simulink library "tqd"  (R2021b)
settings: Solver=VariableStepAuto  StartTime=0.0  StopTime=10.0  RelTol=1e-3
undefined symbols (not defined in the file): ATQD_AfterTqMinGain_X_Deg, ATQD_APSCreepBaseTqD_X_kph, ATQD_APSCreepBaseTqD_Y_Deg, ATQD_APSCreepBaseTqR_X_kph, ATQD_APSCreepBaseTqR_Y_Deg, ATQD_APSCreepIterm_X_kph, ATQD_APSCreepIterm_Y_kph, ATQD_APSCreepPterm_X_kph, ATQD_APSCreepPterm_Y_kph, ATQD_APSDecReq_X_kph, ATQD_APSDecReq_Y_mps2, ATQD_APSDecReqCMD_X_kph, ATQD_APSDecReqTs_X_pct, ATQD_APSDecTimeGain_X_Deg, ATQD_APSDecTimeGain_Y_s, ATQD_APSReqLowSpd_X_Deg, ATQD_AutoHoldReleaseBPS_X_Deg, ATQD_AWDLoadTrqnsGain_X_kg, ATQD_AWDLoadTrqnsGain_Y_pct, ATQD_BOSEnBPSPosn_X_kph, ATQD_BOSMap_X_rpm, ATQD_BOSMap_Y_pct, ATQD_CreepBaseTqD_X_kph, ATQD_CreepBaseTqD_Y_Deg, ATQD_CreepBaseTqR_X_kph, ATQD_CreepBaseTqR_Y_Deg, ATQD_CreepBPSDisPosn_X_Deg, ATQD_CreepBPSDisPosnR_X_Deg, ATQD_CreepBPSEnPosn_X_Deg, ATQD_CreepBPSEnPosnR_X_Deg, ATQD_CreepDeltaTq_X_kph, ATQD_CreepIterm_X_kph, ATQD_CreepIterm_Y_kph, ATQD_CreepItermMaxLimit_X_pct, ATQD_CreepPreloadTime_X_kph, ATQD_CreepPreloadTq_X_kph, ATQD_CreepPreloadTq_Y_s, ATQD_CreepProtTq_X_Deg, ATQD_CreepPterm_X_kph, ATQD_CreepPterm_Y_kph, ATQD_CreepRrTqSpRat_X_rpm, ATQD_CreepRrTqSpRat_Y_Nm, ATQD_CreepTargetSpdD_X_pct, ATQD_CreepTargetSpdR_X_pct, ATQD_ECOTqMapD_X_rpm, ATQD_ECOTqMapD_Y_pct, ATQD_EMTqMapD_X_rpm, ATQD_EMTqMapD_Y_pct, ATQD_EOPDTqMapDCon_X_rpm, ATQD_EOPDTqMapDCon_Y_Deg, ATQD_EscapeModePedTq_X_pct, ATQD_EscapeModePedTq_Y_rpm, ATQD_EscapeModePedTqFr_X_pct, ATQD_EscapeModePedTqFr_Y_rpm, ATQD_EstInitVehWeight_X_c, ATQD_FAfterTqCMDGain_X_rpm, ATQD_FAfterTqCMDGain_Y_pct, ATQD_FrLossMAPLowV_X_rpm, ATQD_FrLossMAPLowV_Y_Nm, ATQD_FrMotActReduce_X_rpm ... (+772)
libraries: simulink x211, hcu_lib x179, tqr x3
(part 21 of 28)

== system tqd/TQD/TorqueDemand/TorqueModule/DriverWhlTqDem/PedalMapWhlTq/Pedal G-Control Mode/Torque Calculation ==
  VTQD_ActAPSPosn_pct : Inport
  VTQD_TqTargetShaftSpd_rpm : Inport  Port=2
  VVMC_LongAcc_Gps : Inport  Port=3
  VINP_VehSpeed_kph : Inport  Port=4
  VTQD_PedAccTqEn_flg : Inport  Port=5
  VTQD_GearActualPosn_enum : Inport  Port=6
  VTQD_CreepPrLoadEnable_flg : Inport  Port=7
  VINP_BrkPedalPos_pct : Inport  Port=8
  VINP_IVIPedalGRegenLim_pct : Inport  Port=9
  VVMC_SmartRegenReq_mps2 : Inport  Port=10
  VINP_IVISmartRegenSW_flg : Inport  Port=11
  VINP_IVICreepOnSW_flg : Inport  Port=12
  VTQD_APSReqTimer_s : Inport  Port=13
  AND{,1..3} (4 alike) : Logic  AllPortsSameDT=off  OutDataTypeStr=boolean
  Add : Sum
  Add1 : Sum  Inputs=+-
  Constant1 : Constant  Value=KTQD_PedAccCMDUpLim_mps2
  Constant10 : Constant  Value=KVMC_GravityValue_mps2
  Constant11 : Constant  Value=KTQD_PedAccDevLowLim_mps2
  Constant12 : Constant  Value=ONE_PERCENT
  Constant13 : Constant  Value=KTQD_PedAccBrkEnPos_pct
  Constant14 : Constant  Value=KTQD_PedAccBrkDeltaTq_Nm
  Constant{6..7,15,21} (4 alike) : Constant  Value=ZERO_INT
  Constant16 : Constant  Value=ZERO_FLOAT
  Constant17 : Constant  Value=KTQD_PedAccARgnEnSpd_kph
  Constant18 : Constant  Value=KTQD_PedAccBrkEnPos_pct
  Constant19 : Constant  Value=KTQD_PedAccDevUpLim_mps2
  Constant2 : Constant  Value=KTQD_PedAccCMDLowLim_mps2
  Constant20 : Constant  Value=KTQD_PedAccARgnEnSpd_kph
  Constant22 : Constant  Value=KTQD_APSReqDelayTime_s
  Constant23 : Constant  Value=KTQD_PedAccCMDLowLim_mps2
  Constant3 : Constant  Value=KTQD_PedAccTqUpLim_Nm
  Constant4 : Constant  Value=KTQD_PedAccTqLowLim_Nm
  Constant5 : Constant  Value=KTQD_PedGControlEnSpd_kph
  Constant8 : Constant  Value=ENUM_GEARACTUALPOSN_D
  Constant9 : Constant  Value=ZERO_FLOAT
  Delay : Delay  DelayLength=1
  Delay1 : Delay  DelayLength=1
  Equal : RelationalOperator  Operator===  OutDataTypeStr=boolean  RndMeth=Simplest
  Equal1 : RelationalOperator  OutDataTypeStr=boolean  RndMeth=Simplest
  MTQD_PedAccBrkTq_Y_Nm : Lookup_n-D  NumberOfTableDimensions=1  BreakpointsForDimension1=ATQD_PedAccBrkTq_X_pct  Table=MTQD_PedAccBrkTq_Y_Nm  InternalRulePriority=Speed  RndMeth=Simplest  InputSameDT=on
  MTQD_PedalAccelCMDWC_Z_mps2 : Lookup_n-D  BreakpointsForDimension1=ATQD_PedalAccelCMD_Y_pct  BreakpointsForDimension2=ATQD_PedalAccelCMD_X_rpm  BreakpointsForDimension3=[5, 7]  Table=MTQD_PedalAccelCMDWC_Z_mps2  ExtrapMethod=Clip  InternalRulePriority=Speed  RndMeth=Simplest  InputSameDT=on
      settings: InputPortMap=u0,u1
  MTQD_PedalAccelCMD_Z_mps2 : Lookup_n-D  BreakpointsForDimension1=ATQD_PedalAccelCMD_Y_pct  BreakpointsForDimension2=ATQD_PedalAccelCMD_X_rpm  BreakpointsForDimension3=[5, 7]  Table=MTQD_PedalAccelCMD_Z_mps2  ExtrapMethod=Clip  InternalRulePriority=Speed  RndMeth=Simplest  InputSameDT=on
      settings: InputPortMap=u0,u1
  MTQD_PedalGDeltaTqIGain_Z_Nm : Lookup_n-D  BreakpointsForDimension1=ATQD_PedalGDeltaTqIGain_Y_mps2  BreakpointsForDimension2=ATQD_PedalGDeltaTqIGain_X_kph  Table=MTQD_PedalGDeltaTqIGain_Z_Nm  InternalRulePriority=Speed  RndMeth=Simplest  InputSameDT=on
      settings: InputPortMap=u0,u1
  Max : MinMax  Function=max  Inputs=2
  OR : Logic  Operator=OR  AllPortsSameDT=off  OutDataTypeStr=boolean
  OR1 : Logic  Operator=OR  AllPortsSameDT=off  OutDataTypeStr=boolean
  Product : Product
  Product1 : Product  Inputs=3
  Relational Operator : RelationalOperator  Operator=<=  OutDataTypeStr=boolean  RndMeth=Simplest
  Relational Operator1 : RelationalOperator  Operator=<=  OutDataTypeStr=boolean  RndMeth=Simplest
  Relational Operator3 : RelationalOperator  OutDataTypeStr=boolean  RndMeth=Simplest
  Relational Operator4 : RelationalOperator  OutDataTypeStr=boolean  RndMeth=Simplest
  Relational Operator5 : RelationalOperator  Operator=>  OutDataTypeStr=boolean  RndMeth=Simplest
  Relational Operator6 : RelationalOperator  OutDataTypeStr=boolean  RndMeth=Simplest
  Relational Operator7 : RelationalOperator  Operator=<=  OutDataTypeStr=boolean  RndMeth=Simplest
  Saturation Dynamic{,1..3} (4 alike) : simulink/Discontinuities/Saturation Dynamic  OutMin=[]  OutMax=[]  OutDataTypeStr=Inherit: Same as second input  OutDataType=fixdt(1, 16)  OutScaling=2^-10  DoSatur=off
  Switch{,1..6} (7 alike) : Switch  Criteria=u2 > Threshold
  VTQD_PedalTqCal_Nm : Outport
  wires:
  Saturation Dynamic1/1 -> MTQD_PedalGDeltaTqIGain_Z_Nm/1  "VTQD_PedalAccDev_mps2"
  [VTQD_PedalAccDeltaTq_Nm] -> Add/1
  Constant11/1 -> Saturation Dynamic1/3
  [VTQD_PedalReqAccel_mps2] -> Add1/1
  [VTQD_ActAPSPosn_pct] -> MTQD_PedalAccelCMD_Z_mps2/1
  [VTQD_TqTargetShaftSpd_rpm] -> MTQD_PedalAccelCMD_Z_mps2/2
  Constant6/1 -> Switch/3
  [VVMC_LongAcc_Gps] -> Product/1
  [VINP_VehSpeed_kph] -> MTQD_PedalGDeltaTqIGain_Z_Nm/2
  Add1/1 -> Saturation Dynamic1/2
  Constant19/1 -> Saturation Dynamic1/1
  Constant10/1 -> Product/2
  Constant1/1 -> Saturation Dynamic2/1
  Delay/1 -> [VTQD_LastPedalTqCal_Nm]  "VTQD_LastPedalTqCal_Nm"
  Product/1 -> Add1/2
  Switch/1 -> Saturation Dynamic/2
  Saturation Dynamic2/1 -> [VTQD_PedalReqAccel_mps2]  "VTQD_PedalReqAccel_mps2"
  [VTQD_LastPedalTqCal_Nm] -> Add/2
  VTQD_ActAPSPosn_pct/1 -> [VTQD_ActAPSPosn_pct]
  VTQD_TqTargetShaftSpd_rpm/1 -> [VTQD_TqTargetShaftSpd_rpm]
  VVMC_LongAcc_Gps/1 -> [VVMC_LongAcc_Gps]
  VINP_VehSpeed_kph/1 -> [VINP_VehSpeed_kph]
  VTQD_PedAccTqEn_flg/1 -> [VTQD_PedAccTqEn_flg]
  [VTQD_PedalTqCal_Nm] -> VTQD_PedalTqCal_Nm/1
  [VINP_VehSpeed_kph] -> Relational Operator/1
  Constant5/1 -> Relational Operator/2
  Relational Operator/1 -> AND/1
  Constant4/1 -> Switch1/3
  Constant7/1 -> Switch1/1
  Switch1/1 -> [VTQD_PedAccTqLowLim_Nm]  "VTQD_PedAccTqLowLim_Nm"
  [VTQD_PedAccTqLowLim_Nm] -> Saturation Dynamic/3
  [VTQD_PedAccTqEn_flg] -> AND1/1
  Equal/1 -> AND1/2
  [VTQD_GearActualPosn_enum] -> Equal/1
  Constant8/1 -> Equal/2
  VTQD_GearActualPosn_enum/1 -> [VTQD_GearActualPosn_enum]
  VTQD_CreepPrLoadEnable_flg/1 -> [VTQD_CreepPrLoadEnable_flg]
  Add/1 -> Switch/1
  [VTQD_PedalReqAccel_mps2] -> Relational Operator1/1
  Relational Operator1/1 -> AND/2
  Constant9/1 -> Relational Operator1/2
  AND/1 -> OR1/1
  OR1/1 -> Switch1/2
  Delay1/1 -> OR1/2
  [VTQD_CreepPrLoadEnable_flg] -> Delay1/1
  VINP_BrkPedalPos_pct/1 -> [VINP_BrkPedalPos_pct]
  [VINP_BrkPedalPos_pct] -> Relational Operator3/1
  Constant13/1 -> Relational Operator3/2
  Switch3/1 -> Switch2/1
  Constant14/1 -> Switch3/1
  [VTQD_LastPedalTqCal_Nm] -> Relational Operator4/1
  Relational Operator4/1 -> Switch3/2
  Constant16/1 -> Switch3/3
  Saturation Dynamic/1 -> [VTQD_PedalTqCal_Nm], Delay/1  "VTQD_PedalTqCal_Nm"
  MTQD_PedalGDeltaTqIGain_Z_Nm/1 -> Switch2/3
  Switch2/1 -> [VTQD_PedalAccDeltaTq_Nm]  "VTQD_PedalAccDeltaTq_Nm"
  AND2/1 -> Switch2/2
  Relational Operator3/1 -> AND2/1
  [VINP_VehSpeed_kph] -> Relational Operator5/1
  Constant17/1 -> Relational Operator5/2
  Relational Operator5/1 -> AND2/2
  Relational Operator7/1 -> AND3/2
  Constant20/1 -> Relational Operator7/2
  [VINP_BrkPedalPos_pct] -> Relational Operator6/1
  Constant18/1 -> Relational Operator6/2
  [VINP_VehSpeed_kph] -> Relational Operator7/1
  Relational Operator6/1 -> AND3/1
  AND3/1 -> Switch4/2
  Constant3/1 -> Switch4/3
  Constant21/1 -> Switch4/1
  Switch4/1 -> [VTQD_PedAccTqUpLim_Nm]  "VTQD_PedAccTqUpLim_Nm"
  [VTQD_PedAccTqUpLim_Nm] -> Saturation Dynamic/1
  [VTQD_PedAccBrkTq_Nm] -> Relational Operator4/2
  MTQD_PedAccBrkTq_Y_Nm/1 -> Saturation Dynamic3/2
  Saturation Dynamic3/1 -> [VTQD_PedAccBrkTq_Nm]  "VTQD_PedAccBrkTq_Nm"
  Constant15/1 -> Saturation Dynamic3/1
  [VTQD_PedAccTqLowLim_Nm] -> Saturation Dynamic3/3
  VINP_IVIPedalGRegenLim_pct/1 -> [VINP_IVIPedalGRegenLim_pct]
  [VINP_IVIPedalGRegenLim_pct] -> MTQD_PedAccBrkTq_Y_Nm/1
  Constant2/1 -> Product1/1
  [VINP_IVIPedalGRegenLim_pct] -> Product1/2
  Constant12/1 -> Product1/3
  Product1/1 -> Max/1
  Max/1 -> Saturation Dynamic2/3
  Switch5/1 -> Max/2
  [VVMC_SmartRegenReq_mps2] -> Switch5/1
  Constant23/1 -> Switch5/3
  [VINP_IVISmartRegenSW_flg] -> Switch5/2
  VVMC_SmartRegenReq_mps2/1 -> [VVMC_SmartRegenReq_mps2]
  VINP_IVISmartRegenSW_flg/1 -> [VINP_IVISmartRegenSW_flg]
  MTQD_PedalAccelCMD_Z_mps2/1 -> [VTQD_PedalAccelCMD_mps2]  "VTQD_PedalAccelCMD_mps2"
  MTQD_PedalAccelCMDWC_Z_mps2/1 -> [VTQD_PedalAccelCMDWC_mps2]  "VTQD_PedalAccelCMDWC_mps2"
  [VTQD_TqTargetShaftSpd_rpm] -> MTQD_PedalAccelCMDWC_Z_mps2/2
  [VTQD_ActAPSPosn_pct] -> MTQD_PedalAccelCMDWC_Z_mps2/1
  VINP_IVICreepOnSW_flg/1 -> [VINP_IVICreepOnSW_flg]
  Switch6/1 -> Saturation Dynamic2/2
  [VINP_IVICreepOnSW_flg] -> Switch6/2
  [VTQD_PedalAccelCMD_mps2] -> Switch6/3
  [VTQD_PedalAccelCMDWC_mps2] -> Switch6/1
  VTQD_APSReqTimer_s/1 -> [VTQD_APSReqTimer_s]
  OR/1 -> Switch/2
  AND1/1 -> OR/1
  Equal1/1 -> OR/2
  [VTQD_APSReqTimer_s] -> Equal1/1
  Constant22/1 -> Equal1/2

== system tqd/TQD/TorqueDemand/Signal_convert/SWC2_Subsystem/Big Mike Combo/Combo Key Detection/DiagnosisOff Mode/Key1 ==
  VSCP_ComboKeyCMD_enum : Inport
  VSCP_ComboKeyEn_flg : Inport  Port=2
  VSCP_ComboKeyReset_flg : Inport  Port=3
  AND : Logic  Inputs=3  AllPortsSameDT=off  OutDataTypeStr=boolean
  Constant1 : Constant  Value=KTQD_DiagnosisOff1_enum
  Constant2 : Constant  Value=ENUM_COMBOKEY_NONE
  Constant4 : Constant  Value=ENUM_COMBOKEY_NONE
  Data Type Conversion : DataTypeConversion  OutDataTypeStr=uint8
  Delay : Delay  DelayLength=1
  Delay1 : Delay  DelayLength=1
  Detect Change : simulink/Logic and Bit Operations/Detect Change  vinit=0  OutDataTypeStr=boolean
  Detect Increase : simulink/Logic and Bit Operations/Detect Increase  vinit=0.0  OutDataTypeStr=boolean
  Equal : RelationalOperator  Operator===  OutDataTypeStr=boolean  RndMeth=Simplest
  Equal1 : RelationalOperator  Operator=~=  OutDataTypeStr=boolean  RndMeth=Simplest
  Equal2 : RelationalOperator  Operator===  OutDataTypeStr=boolean  RndMeth=Simplest
  If : If  NumInputs=2  IfExpression=u1 ~=0  ElseIfExpressions=u2 ~= 0
  Maintain : Subsystem  TreatAsAtomicUnit=on
  Merge : Merge  Inputs=3
  OR : Logic  Operator=OR  AllPortsSameDT=off  OutDataTypeStr=boolean
  Reset : Subsystem  TreatAsAtomicUnit=on
  Write : Subsystem  TreatAsAtomicUnit=on
  VSCP_ComboKey1_enum : Outport
  VSCP_Key1Pass_flg : Outport  Port=2
  wires:
  Data Type Conversion/1 -> [VSCP_ComboKey1_enum]  "VTQD_DiagnosisOff1_enum"
  Delay1/1 -> Maintain/1(Input)
  [VSCP_ComboKey1_enum] -> Delay1/1
  [VSCP_Key1Pass_flg] -> VSCP_Key1Pass_flg/1
  [VSCP_ComboKey1_enum] -> VSCP_ComboKey1_enum/1
  VSCP_ComboKeyEn_flg/1 -> [VSCP_ComboKeyEn_flg]
  VSCP_ComboKeyReset_flg/1 -> [VSCP_ComboKeyReset_flg]
  VSCP_ComboKeyCMD_enum/1 -> [VSCP_ComboKeyCMD_enum]
  Equal/1 -> [VSCP_Key1Pass_flg]  "VTQD_DiagnosisOff1Pass_flg"
  Constant1/1 -> Equal/2
  [VSCP_ComboKey1_enum] -> Equal/1
  If/2 -> Write/Action
  Write/1(WriteCMD) -> Merge/2
  If/1 -> Reset/Action
  Detect Increase/1 -> OR/1
  AND/1 -> [VSCP_WriteComboCMD_flg]  "VSCP_WriteComboCMD_flg"
  [VSCP_ComboKeyCMD_enum] -> Write/1(Input)
  [VSCP_ComboKeyCMD_enum] -> Detect Change/1
  [VSCP_ResetComboKey_flg] -> If/1
  [VSCP_ComboKeyEn_flg] -> Detect Increase/1
  Detect Change/1 -> AND/1
  Maintain/1(KeepKey1) -> Merge/3
  Constant4/1 -> Equal1/2
  If/3 -> Maintain/Action
  Delay/1 -> Equal2/1
  Merge/1 -> Data Type Conversion/1
  Reset/1(ResetToZero) -> Merge/1
  Equal2/1 -> AND/3
  Constant2/1 -> Equal2/2
  Equal1/1 -> AND/2
  [VSCP_ComboKey1_enum] -> Delay/1
  [VSCP_ComboKeyReset_flg] -> OR/2
  [VSCP_ComboKeyCMD_enum] -> Equal1/1
  [VSCP_WriteComboCMD_flg] -> If/2
  OR/1 -> [VSCP_ResetComboKey_flg]  "VSCP_ResetComboKey_flg"

== system tqd/TQD/TorqueDemand/Signal_convert/SWC2_Subsystem/Big Mike Combo/Combo Key Detection/DiagnosisOff Mode/Key2 ==
  VSCP_ComboKeyCMD_enum : Inport
  VSCP_ComboKeyEn_flg : Inport  Port=2
  VSCP_ComboKeyReset_flg : Inport  Port=3
  VSCP_ComboKey1_enum : Inport  Port=4
  AND : Logic  Inputs=4  AllPortsSameDT=off  OutDataTypeStr=boolean
  Constant1 : Constant  Value=KTQD_DiagnosisOff2_enum
  Constant2 : Constant  Value=ENUM_COMBOKEY_NONE
  Constant3 : Constant  Value=ENUM_COMBOKEY_NONE
  Constant4 : Constant  Value=ENUM_COMBOKEY_NONE  OutDataTypeStr=uint8
  Data Type Conversion : DataTypeConversion  OutDataTypeStr=uint8
  Delay : Delay  DelayLength=1
  Delay1 : Delay  DelayLength=1
  Delay2 : Delay  DelayLength=1
  Detect Change : simulink/Logic and Bit Operations/Detect Change  vinit=0  OutDataTypeStr=boolean
  Detect Increase : simulink/Logic and Bit Operations/Detect Increase  vinit=0.0  OutDataTypeStr=boolean
  Equal : RelationalOperator  Operator===  OutDataTypeStr=boolean  RndMeth=Simplest
  Equal1 : RelationalOperator  Operator=~=  OutDataTypeStr=boolean  RndMeth=Simplest
  Equal2 : RelationalOperator  Operator=~=  OutDataTypeStr=boolean  RndMeth=Simplest
  Equal3 : RelationalOperator  Operator===  OutDataTypeStr=boolean  RndMeth=Simplest
  If : If  NumInputs=2  IfExpression=u1 ~=0  ElseIfExpressions=u2 ~= 0
  Maintain : Subsystem  TreatAsAtomicUnit=on
  Merge : Merge  Inputs=3
  OR : Logic  Operator=OR  AllPortsSameDT=off  OutDataTypeStr=boolean
  Reset : Subsystem  TreatAsAtomicUnit=on
  Write : Subsystem  TreatAsAtomicUnit=on
  VSCP_ComboKey2_enum : Outport
  VSCP_Key2Pass_flg : Outport  Port=2
  wires:
  Data Type Conversion/1 -> [VSCP_ComboKey2_enum]  "VTQD_DiagnosisOff2_enum"
  [VSCP_ComboKey2_enum] -> Delay2/1
  Delay2/1 -> Maintain/1(Input)
  Equal3/1 -> AND/4
  Delay1/1 -> Equal3/1
  Constant3/1 -> Equal3/2
  [VSCP_ComboKey2_enum] -> Delay1/1
  VSCP_ComboKey1_enum/1 -> [VSCP_ComboKey1_enum]
  OR/1 -> [VSCP_ResetComboKey_flg]  "VSCP_ResetComboKey_flg"
  [VSCP_WriteComboCMD_flg] -> If/2
  [VSCP_ComboKeyCMD_enum] -> Equal1/1
  [VSCP_ComboKeyReset_flg] -> OR/2
  [VSCP_ComboKey1_enum] -> Delay/1
  Equal1/1 -> AND/2
  Constant2/1 -> Equal2/2
  Equal2/1 -> AND/3
  Reset/1(ResetToZero) -> Merge/1
  Merge/1 -> Data Type Conversion/1
  Delay/1 -> Equal2/1
  If/3 -> Maintain/Action
  Constant4/1 -> Equal1/2
  Maintain/1(KeepKey2) -> Merge/3
  Detect Change/1 -> AND/1
  [VSCP_ComboKeyEn_flg] -> Detect Increase/1
  [VSCP_ResetComboKey_flg] -> If/1
  [VSCP_ComboKeyCMD_enum] -> Detect Change/1
  [VSCP_ComboKeyCMD_enum] -> Write/1(Input)
  AND/1 -> [VSCP_WriteComboCMD_flg]  "VSCP_WriteComboCMD_flg"
  Detect Increase/1 -> OR/1
  If/1 -> Reset/Action
  Write/1(WriteCMD) -> Merge/2
  If/2 -> Write/Action
  [VSCP_ComboKey2_enum] -> Equal/1
  Constant1/1 -> Equal/2
  Equal/1 -> [VSCP_Key2Pass_flg]  "VTQD_DiagnosisOff2Pass_flg"
  VSCP_ComboKeyCMD_enum/1 -> [VSCP_ComboKeyCMD_enum]
  VSCP_ComboKeyReset_flg/1 -> [VSCP_ComboKeyReset_flg]
  VSCP_ComboKeyEn_flg/1 -> [VSCP_ComboKeyEn_flg]
  [VSCP_ComboKey2_enum] -> VSCP_ComboKey2_enum/1
  [VSCP_Key2Pass_flg] -> VSCP_Key2Pass_flg/1

== system tqd/TQD/TorqueDemand/Signal_convert/SWC2_Subsystem/Big Mike Combo/Combo Key Detection/DiagnosisOff Mode/Key3 ==
  VSCP_ComboKeyCMD_enum : Inport
  VSCP_ComboKeyEn_flg : Inport  Port=2
  VSCP_ComboKeyReset_flg : Inport  Port=3
  VSCP_ComboKey2_enum : Inport  Port=4
  AND : Logic  Inputs=4  AllPortsSameDT=off  OutDataTypeStr=boolean
  Constant1 : Constant  Value=KTQD_DiagnosisOff3_enum
  Constant2 : Constant  Value=ENUM_COMBOKEY_NONE
  Constant3 : Constant  Value=ENUM_COMBOKEY_NONE
  Constant4 : Constant  Value=ENUM_COMBOKEY_NONE
  Data Type Conversion : DataTypeConversion  OutDataTypeStr=uint8
  Delay : Delay  DelayLength=1
  Delay1 : Delay  DelayLength=1
  Delay2 : Delay  DelayLength=1
  Detect Change : simulink/Logic and Bit Operations/Detect Change  vinit=0  OutDataTypeStr=boolean
  Detect Increase : simulink/Logic and Bit Operations/Detect Increase  vinit=0.0  OutDataTypeStr=boolean
  Equal : RelationalOperator  Operator===  OutDataTypeStr=boolean  RndMeth=Simplest
  Equal1 : RelationalOperator  Operator=~=  OutDataTypeStr=boolean  RndMeth=Simplest
  Equal2 : RelationalOperator  Operator=~=  OutDataTypeStr=boolean  RndMeth=Simplest
  Equal3 : RelationalOperator  Operator===  OutDataTypeStr=boolean  RndMeth=Simplest
  If : If  NumInputs=2  IfExpression=u1 ~=0  ElseIfExpressions=u2 ~= 0
  Maintain : Subsystem  TreatAsAtomicUnit=on
  Merge : Merge  Inputs=3
  OR : Logic  Operator=OR  AllPortsSameDT=off  OutDataTypeStr=boolean
  Reset : Subsystem  TreatAsAtomicUnit=on
  Write : Subsystem  TreatAsAtomicUnit=on
  VSCP_ComboKey3_enum : Outport
  VSCP_Key3Pass_flg : Outport  Port=2
  wires:
  Data Type Conversion/1 -> [VSCP_ComboKey3_enum]  "VTQD_DiagnosisOff3_enum"
  [VSCP_ComboKey3_enum] -> Delay2/1
  Delay2/1 -> Maintain/1(Input)
  [VSCP_ComboKey3_enum] -> Delay1/1
  Constant3/1 -> Equal3/2
  Equal3/1 -> AND/4
  Delay1/1 -> Equal3/1
  [VSCP_Key3Pass_flg] -> VSCP_Key3Pass_flg/1
  [VSCP_ComboKey3_enum] -> Equal/1
  [VSCP_ComboKey3_enum] -> VSCP_ComboKey3_enum/1
  VSCP_ComboKeyEn_flg/1 -> [VSCP_ComboKeyEn_flg]
  VSCP_ComboKeyReset_flg/1 -> [VSCP_ComboKeyReset_flg]
  VSCP_ComboKeyCMD_enum/1 -> [VSCP_ComboKeyCMD_enum]
  Equal/1 -> [VSCP_Key3Pass_flg]  "VTQD_DiagnosisOff3Pass_flg"
  Constant1/1 -> Equal/2
  If/2 -> Write/Action
  Write/1(WriteCMD) -> Merge/2
  If/1 -> Reset/Action
  Detect Increase/1 -> OR/1
  AND/1 -> [VSCP_WriteComboCMD_flg]  "VSCP_WriteComboCMD_flg"
  [VSCP_ComboKeyCMD_enum] -> Write/1(Input)
  [VSCP_ComboKeyCMD_enum] -> Detect Change/1
  [VSCP_ResetComboKey_flg] -> If/1
  [VSCP_ComboKeyEn_flg] -> Detect Increase/1
  Detect Change/1 -> AND/1
  Maintain/1(KeepKey3) -> Merge/3
  Constant4/1 -> Equal1/2
  If/3 -> Maintain/Action
  Delay/1 -> Equal2/1
  Merge/1 -> Data Type Conversion/1
  Reset/1(ResetToZero) -> Merge/1
  Equal2/1 -> AND/3
  Constant2/1 -> Equal2/2
  Equal1/1 -> AND/2
  [VSCP_ComboKey2_enum] -> Delay/1
  [VSCP_ComboKeyReset_flg] -> OR/2
  [VSCP_ComboKeyCMD_enum] -> Equal1/1
  [VSCP_WriteComboCMD_flg] -> If/2
  OR/1 -> [VSCP_ResetComboKey_flg]  "VSCP_ResetComboKey_flg"
  VSCP_ComboKey2_enum/1 -> [VSCP_ComboKey2_enum]

== system tqd/TQD/TorqueDemand/Signal_convert/SWC2_Subsystem/Big Mike Combo/Combo Key Detection/DiagnosisOff Mode/Key4 ==
  VSCP_ComboKeyCMD_enum : Inport
  VSCP_ComboKeyEn_flg : Inport  Port=2
  VSCP_ComboKeyReset_flg : Inport  Port=3
  VSCP_ComboKey3_enum : Inport  Port=4
  AND : Logic  Inputs=4  AllPortsSameDT=off  OutDataTypeStr=boolean
  Constant1 : Constant  Value=KTQD_DiagnosisOff4_enum
  Constant2 : Constant  Value=ENUM_COMBOKEY_NONE
  Constant3 : Constant  Value=ENUM_COMBOKEY_NONE
  Constant4 : Constant  Value=ENUM_COMBOKEY_NONE
  Data Type Conversion : DataTypeConversion  OutDataTypeStr=uint8
  Delay : Delay  DelayLength=1
  Delay1 : Delay  DelayLength=1
  Delay2 : Delay  DelayLength=1
  Detect Change : simulink/Logic and Bit Operations/Detect Change  vinit=0  OutDataTypeStr=boolean
  Detect Increase : simulink/Logic and Bit Operations/Detect Increase  vinit=0.0  OutDataTypeStr=boolean
  Equal : RelationalOperator  Operator===  OutDataTypeStr=boolean  RndMeth=Simplest
  Equal1 : RelationalOperator  Operator=~=  OutDataTypeStr=boolean  RndMeth=Simplest
  Equal2 : RelationalOperator  Operator=~=  OutDataTypeStr=boolean  RndMeth=Simplest
  Equal3 : RelationalOperator  Operator===  OutDataTypeStr=boolean  RndMeth=Simplest
  If : If  NumInputs=2  IfExpression=u1 ~=0  ElseIfExpressions=u2 ~= 0
  Maintain : Subsystem  TreatAsAtomicUnit=on
  Merge : Merge  Inputs=3
  OR : Logic  Operator=OR  AllPortsSameDT=off  OutDataTypeStr=boolean
  Reset : Subsystem  TreatAsAtomicUnit=on
  Write : Subsystem  TreatAsAtomicUnit=on
  VSCP_ComboKey4_enum : Outport
  VSCP_Key4Pass_flg : Outport  Port=2
  wires:
  Data Type Conversion/1 -> [VSCP_ComboKey4_enum]  "VTQD_DiagnosisOff4_enum"
  Delay2/1 -> Maintain/1(Input)
  [VSCP_ComboKey4_enum] -> Delay2/1
  [VSCP_ComboKey4_enum] -> VSCP_ComboKey4_enum/1
  [VSCP_Key4Pass_flg] -> VSCP_Key4Pass_flg/1
  Equal3/1 -> AND/4
  Delay1/1 -> Equal3/1
  Constant3/1 -> Equal3/2
  [VSCP_ComboKey4_enum] -> Delay1/1
  VSCP_ComboKey3_enum/1 -> [VSCP_ComboKey3_enum]
  OR/1 -> [VSCP_ResetComboKey_flg]  "VSCP_ResetComboKey_flg"
  [VSCP_WriteComboCMD_flg] -> If/2
  [VSCP_ComboKeyCMD_enum] -> Equal1/1
  [VSCP_ComboKeyReset_flg] -> OR/2
  [VSCP_ComboKey3_enum] -> Delay/1
  Equal1/1 -> AND/2
  Constant2/1 -> Equal2/2
  Equal2/1 -> AND/3
  Reset/1(ResetToZero) -> Merge/1
  Merge/1 -> Data Type Conversion/1
  Delay/1 -> Equal2/1
  If/3 -> Maintain/Action
  Constant4/1 -> Equal1/2
  Maintain/1(KeepKey4) -> Merge/3
  Detect Change/1 -> AND/1
  [VSCP_ComboKeyEn_flg] -> Detect Increase/1
  [VSCP_ResetComboKey_flg] -> If/1
  [VSCP_ComboKeyCMD_enum] -> Detect Change/1
  [VSCP_ComboKeyCMD_enum] -> Write/1(Input)
  AND/1 -> [VSCP_WriteComboCMD_flg]  "VSCP_WriteComboCMD_flg"
  Detect Increase/1 -> OR/1
  If/1 -> Reset/Action
  Write/1(WriteCMD) -> Merge/2
  If/2 -> Write/Action
  Constant1/1 -> Equal/2
  Equal/1 -> [VSCP_Key4Pass_flg]  "VTQD_DiagnosisOff4Pass_flg"
  VSCP_ComboKeyCMD_enum/1 -> [VSCP_ComboKeyCMD_enum]
  VSCP_ComboKeyReset_flg/1 -> [VSCP_ComboKeyReset_flg]
  VSCP_ComboKeyEn_flg/1 -> [VSCP_ComboKeyEn_flg]
  [VSCP_ComboKey4_enum] -> Equal/1

== system tqd/TQD/TorqueDemand/Signal_convert/SWC2_Subsystem/Big Mike Combo/Combo Key Detection/DiagnosisOff Mode/Key5 ==
  VSCP_ComboKeyCMD_enum : Inport
  VSCP_ComboKeyEn_flg : Inport  Port=2
  VSCP_ComboKeyReset_flg : Inport  Port=3
  VSCP_ComboKey4_enum : Inport  Port=4
  AND : Logic  Inputs=4  AllPortsSameDT=off  OutDataTypeStr=boolean
  Constant1 : Constant  Value=KTQD_DiagnosisOff5_enum
  Constant2 : Constant  Value=ENUM_COMBOKEY_NONE
  Constant3 : Constant  Value=ENUM_COMBOKEY_NONE
  Constant4 : Constant  Value=ENUM_COMBOKEY_NONE
  Data Type Conversion : DataTypeConversion  OutDataTypeStr=uint8
  Delay : Delay  DelayLength=1
  Delay1 : Delay  DelayLength=1
  Delay2 : Delay  DelayLength=1
  Detect Change : simulink/Logic and Bit Operations/Detect Change  vinit=0  OutDataTypeStr=boolean
  Detect Increase : simulink/Logic and Bit Operations/Detect Increase  vinit=0.0  OutDataTypeStr=boolean
  Equal : RelationalOperator  Operator===  OutDataTypeStr=boolean  RndMeth=Simplest
  Equal1 : RelationalOperator  Operator=~=  OutDataTypeStr=boolean  RndMeth=Simplest
  Equal2 : RelationalOperator  Operator=~=  OutDataTypeStr=boolean  RndMeth=Simplest
  Equal3 : RelationalOperator  Operator===  OutDataTypeStr=boolean  RndMeth=Simplest
  If : If  NumInputs=2  IfExpression=u1 ~=0  ElseIfExpressions=u2 ~= 0
  Maintain : Subsystem  TreatAsAtomicUnit=on
  Merge : Merge  Inputs=3
  OR : Logic  Operator=OR  AllPortsSameDT=off  OutDataTypeStr=boolean
  Reset : Subsystem  TreatAsAtomicUnit=on
  Write : Subsystem  TreatAsAtomicUnit=on
  VSCP_ComboKey5_enum : Outport
  VSCP_Key5Pass_flg : Outport  Port=2
  wires:
  Data Type Conversion/1 -> [VSCP_ComboKey5_enum]  "VTQD_DiagnosisOff5_enum"
  Delay2/1 -> Maintain/1(Input)
  [VSCP_ComboKey5_enum] -> Delay2/1
  [VSCP_ComboKey5_enum] -> VSCP_ComboKey5_enum/1
  [VSCP_ComboKey5_enum] -> Equal/1
  VSCP_ComboKeyEn_flg/1 -> [VSCP_ComboKeyEn_flg]
  VSCP_ComboKeyReset_flg/1 -> [VSCP_ComboKeyReset_flg]
  VSCP_ComboKeyCMD_enum/1 -> [VSCP_ComboKeyCMD_enum]
  Equal/1 -> [VSCP_Key5Pass_flg]  "VTQD_DiagnosisOff5Pass_flg"
  Constant1/1 -> Equal/2
  If/2 -> Write/Action
  Write/1(WriteCMD) -> Merge/2
  If/1 -> Reset/Action
  Detect Increase/1 -> OR/1
  AND/1 -> [VSCP_WriteComboCMD_flg]  "VSCP_WriteComboCMD_flg"
  [VSCP_ComboKeyCMD_enum] -> Write/1(Input)
  [VSCP_ComboKeyCMD_enum] -> Detect Change/1
  [VSCP_ResetComboKey_flg] -> If/1
  [VSCP_ComboKeyEn_flg] -> Detect Increase/1
  Detect Change/1 -> AND/1
  Maintain/1(KeepKey5) -> Merge/3
  Constant4/1 -> Equal1/2
  If/3 -> Maintain/Action
  Delay/1 -> Equal2/1
  Merge/1 -> Data Type Conversion/1
  Reset/1(ResetToZero) -> Merge/1
  Equal2/1 -> AND/3
  Constant2/1 -> Equal2/2
  Equal1/1 -> AND/2
  [VSCP_ComboKey4_enum] -> Delay/1
  [VSCP_ComboKeyReset_flg] -> OR/2
  [VSCP_ComboKeyCMD_enum] -> Equal1/1
  [VSCP_WriteComboCMD_flg] -> If/2
  OR/1 -> [VSCP_ResetComboKey_flg]  "VSCP_ResetComboKey_flg"
  VSCP_ComboKey4_enum/1 -> [VSCP_ComboKey4_enum]
  [VSCP_ComboKey5_enum] -> Delay1/1
  Constant3/1 -> Equal3/2
  Delay1/1 -> Equal3/1
  Equal3/1 -> AND/4
  [VSCP_Key5Pass_flg] -> VSCP_Key5Pass_flg/1

== system tqd/TQD/TorqueDemand/Signal_convert/SWC2_Subsystem/Big Mike Combo/Combo Key Detection/DiagnosisOff Mode/Key6 ==
  VSCP_ComboKeyCMD_enum : Inport
  VSCP_ComboKeyEn_flg : Inport  Port=2
  VSCP_ComboKeyReset_flg : Inport  Port=3
  VSCP_ComboKey5_enum : Inport  Port=4
  AND : Logic  Inputs=4  AllPortsSameDT=off  OutDataTypeStr=boolean
  Constant1 : Constant  Value=KTQD_DiagnosisOff6_enum
  Constant2 : Constant  Value=ENUM_COMBOKEY_NONE
  Constant3 : Constant  Value=ENUM_COMBOKEY_NONE
  Constant4 : Constant  Value=ENUM_COMBOKEY_NONE
  Data Type Conversion : DataTypeConversion  OutDataTypeStr=uint8
  Delay : Delay  DelayLength=1
  Delay1 : Delay  DelayLength=1
  Delay2 : Delay  DelayLength=1
  Detect Change : simulink/Logic and Bit Operations/Detect Change  vinit=0  OutDataTypeStr=boolean
  Detect Increase : simulink/Logic and Bit Operations/Detect Increase  vinit=0.0  OutDataTypeStr=boolean
  Equal : RelationalOperator  Operator===  OutDataTypeStr=boolean  RndMeth=Simplest
  Equal1 : RelationalOperator  Operator=~=  OutDataTypeStr=boolean  RndMeth=Simplest
  Equal2 : RelationalOperator  Operator=~=  OutDataTypeStr=boolean  RndMeth=Simplest
  Equal3 : RelationalOperator  Operator===  OutDataTypeStr=boolean  RndMeth=Simplest
  If : If  NumInputs=2  IfExpression=u1 ~=0  ElseIfExpressions=u2 ~= 0
  Maintain : Subsystem  TreatAsAtomicUnit=on
  Merge : Merge  Inputs=3
  OR : Logic  Operator=OR  AllPortsSameDT=off  OutDataTypeStr=boolean
  Reset : Subsystem  TreatAsAtomicUnit=on
  Write : Subsystem  TreatAsAtomicUnit=on
  VSCP_ComboKey6_enum : Outport
  VSCP_Key6Pass_flg : Outport  Port=2
  wires:
  Data Type Conversion/1 -> [VSCP_ComboKey6_enum]  "VTQD_DiagnosisOff6_enum"
  [VSCP_ComboKey6_enum] -> Delay2/1
  Delay2/1 -> Maintain/1(Input)
  [VSCP_Key6Pass_flg] -> VSCP_Key6Pass_flg/1
  Equal3/1 -> AND/4
  Delay1/1 -> Equal3/1
  Constant3/1 -> Equal3/2
  [VSCP_ComboKey6_enum] -> Delay1/1
  VSCP_ComboKey5_enum/1 -> [VSCP_ComboKey5_enum]
  OR/1 -> [VSCP_ResetComboKey_flg]  "VSCP_ResetComboKey_flg"
  [VSCP_WriteComboCMD_flg] -> If/2
  [VSCP_ComboKeyCMD_enum] -> Equal1/1
  [VSCP_ComboKeyReset_flg] -> OR/2
  [VSCP_ComboKey5_enum] -> Delay/1
  Equal1/1 -> AND/2
  Constant2/1 -> Equal2/2
  Equal2/1 -> AND/3
  Reset/1(ResetToZero) -> Merge/1
  Merge/1 -> Data Type Conversion/1
  Delay/1 -> Equal2/1
  If/3 -> Maintain/Action
  Constant4/1 -> Equal1/2
  Maintain/1(KeepKey6) -> Merge/3
  Detect Change/1 -> AND/1
  [VSCP_ComboKeyEn_flg] -> Detect Increase/1
  [VSCP_ResetComboKey_flg] -> If/1
  [VSCP_ComboKeyCMD_enum] -> Detect Change/1
  [VSCP_ComboKeyCMD_enum] -> Write/1(Input)
  AND/1 -> [VSCP_WriteComboCMD_flg]  "VSCP_WriteComboCMD_flg"
  Detect Increase/1 -> OR/1
  If/1 -> Reset/Action
  Write/1(WriteCMD) -> Merge/2
  If/2 -> Write/Action
  Constant1/1 -> Equal/2
  Equal/1 -> [VSCP_Key6Pass_flg]  "VTQD_DiagnosisOff6Pass_flg"
  VSCP_ComboKeyCMD_enum/1 -> [VSCP_ComboKeyCMD_enum]
  VSCP_ComboKeyReset_flg/1 -> [VSCP_ComboKeyReset_flg]
  VSCP_ComboKeyEn_flg/1 -> [VSCP_ComboKeyEn_flg]
  [VSCP_ComboKey6_enum] -> Equal/1
  [VSCP_ComboKey6_enum] -> VSCP_ComboKey6_enum/1

== system tqd/TQD/TorqueDemand/Signal_convert/SWC2_Subsystem/Big Mike Combo/Combo Key Detection/DiagnosisOff Mode/Key7 ==
  VSCP_ComboKeyCMD_enum : Inport
  VSCP_ComboKeyEn_flg : Inport  Port=2
  VSCP_ComboKeyReset_flg : Inport  Port=3
  VSCP_ComboKey6_enum : Inport  Port=4
  AND : Logic  Inputs=4  AllPortsSameDT=off  OutDataTypeStr=boolean
  Constant1 : Constant  Value=KTQD_DiagnosisOff7_enum
  Constant2 : Constant  Value=ENUM_COMBOKEY_NONE  OutDataTypeStr=uint8
  Constant3 : Constant  Value=ENUM_COMBOKEY_NONE
  Constant4 : Constant  Value=ENUM_COMBOKEY_NONE  OutDataTypeStr=uint8
  Data Type Conversion : DataTypeConversion  OutDataTypeStr=uint8
  Delay : Delay  DelayLength=1
  Delay1 : Delay  DelayLength=1
  Delay2 : Delay  DelayLength=1
  Detect Change : simulink/Logic and Bit Operations/Detect Change  vinit=0  OutDataTypeStr=boolean
  Detect Increase : simulink/Logic and Bit Operations/Detect Increase  vinit=0.0  OutDataTypeStr=boolean
  Equal : RelationalOperator  Operator===  OutDataTypeStr=boolean  RndMeth=Simplest
  Equal1 : RelationalOperator  Operator=~=  OutDataTypeStr=boolean  RndMeth=Simplest
  Equal2 : RelationalOperator  Operator=~=  OutDataTypeStr=boolean  RndMeth=Simplest
  Equal3 : RelationalOperator  Operator===  OutDataTypeStr=boolean  RndMeth=Simplest
  If : If  NumInputs=2  IfExpression=u1 ~=0  ElseIfExpressions=u2 ~= 0
  Maintain : Subsystem  TreatAsAtomicUnit=on
  Merge : Merge  Inputs=3
  OR : Logic  Operator=OR  AllPortsSameDT=off  OutDataTypeStr=boolean
  Reset : Subsystem  TreatAsAtomicUnit=on
  Write : Subsystem  TreatAsAtomicUnit=on
  VSCP_ComboKey7_enum : Outport
  VSCP_Key7Pass_flg : Outport  Port=2
  wires:
  Data Type Conversion/1 -> [VSCP_ComboKey7_enum]  "VTQD_DiagnosisOff7_enum"
  Delay2/1 -> Maintain/1(Input)
  [VSCP_ComboKey7_enum] -> Delay2/1
  [VSCP_ComboKey7_enum] -> VSCP_ComboKey7_enum/1
  [VSCP_ComboKey7_enum] -> Equal/1
  VSCP_ComboKeyEn_flg/1 -> [VSCP_ComboKeyEn_flg]
  VSCP_ComboKeyReset_flg/1 -> [VSCP_ComboKeyReset_flg]
  VSCP_ComboKeyCMD_enum/1 -> [VSCP_ComboKeyCMD_enum]
  Equal/1 -> [VSCP_Key7Pass_flg]  "VTQD_DiagnosisOff7Pass_flg"
  Constant1/1 -> Equal/2
  If/2 -> Write/Action
  Write/1(WriteCMD) -> Merge/2
  If/1 -> Reset/Action
  Detect Increase/1 -> OR/1
  AND/1 -> [VSCP_WriteComboCMD_flg]  "VSCP_WriteComboCMD_flg"
  [VSCP_ComboKeyCMD_enum] -> Write/1(Input)
  [VSCP_ComboKeyCMD_enum] -> Detect Change/1
  [VSCP_ResetComboKey_flg] -> If/1
  [VSCP_ComboKeyEn_flg] -> Detect Increase/1
  Detect Change/1 -> AND/1
  Maintain/1(KeepKey7) -> Merge/3
  Constant4/1 -> Equal1/2
  If/3 -> Maintain/Action
  Delay/1 -> Equal2/1
  Merge/1 -> Data Type Conversion/1
  Reset/1(ResetToZero) -> Merge/1
  Equal2/1 -> AND/3
  Constant2/1 -> Equal2/2
  Equal1/1 -> AND/2
  [VSCP_ComboKey6_enum] -> Delay/1
  [VSCP_ComboKeyReset_flg] -> OR/2
  [VSCP_ComboKeyCMD_enum] -> Equal1/1
  [VSCP_WriteComboCMD_flg] -> If/2
  OR/1 -> [VSCP_ResetComboKey_flg]  "VSCP_ResetComboKey_flg"
  VSCP_ComboKey6_enum/1 -> [VSCP_ComboKey6_enum]
  [VSCP_ComboKey7_enum] -> Delay1/1
  Constant3/1 -> Equal3/2
  Delay1/1 -> Equal3/1
  Equal3/1 -> AND/4
  [VSCP_Key7Pass_flg] -> VSCP_Key7Pass_flg/1

== system tqd/TQD/TorqueDemand/Signal_convert/SWC2_Subsystem/Big Mike Combo/Combo Key Detection/DiagnosisOff Mode/Key8 ==
  VSCP_ComboKeyCMD_enum : Inport
  VSCP_ComboKeyEn_flg : Inport  Port=2
  VSCP_ComboKeyReset_flg : Inport  Port=3
  VSCP_ComboKey7_enum : Inport  Port=4
  AND : Logic  Inputs=4  AllPortsSameDT=off  OutDataTypeStr=boolean
  Constant1 : Constant  Value=KTQD_DiagnosisOff8_enum
  Constant2 : Constant  Value=ENUM_COMBOKEY_NONE
  Constant3 : Constant  Value=ENUM_COMBOKEY_NONE
  Constant4 : Constant  Value=ENUM_COMBOKEY_NONE
  Data Type Conversion : DataTypeConversion  OutDataTypeStr=uint8
  Delay : Delay  DelayLength=1
  Delay1 : Delay  DelayLength=1
  Delay2 : Delay  DelayLength=1
  Detect Change : simulink/Logic and Bit Operations/Detect Change  vinit=0  OutDataTypeStr=boolean
  Detect Increase : simulink/Logic and Bit Operations/Detect Increase  vinit=0.0  OutDataTypeStr=boolean
  Equal : RelationalOperator  Operator===  OutDataTypeStr=boolean  RndMeth=Simplest
  Equal1 : RelationalOperator  Operator=~=  OutDataTypeStr=boolean  RndMeth=Simplest
  Equal2 : RelationalOperator  Operator=~=  OutDataTypeStr=boolean  RndMeth=Simplest
  Equal3 : RelationalOperator  Operator===  OutDataTypeStr=boolean  RndMeth=Simplest
  If : If  NumInputs=2  IfExpression=u1 ~=0  ElseIfExpressions=u2 ~= 0
  Maintain : Subsystem  TreatAsAtomicUnit=on
  Merge : Merge  Inputs=3
  OR : Logic  Operator=OR  AllPortsSameDT=off  OutDataTypeStr=boolean
  Reset : Subsystem  TreatAsAtomicUnit=on
  Write : Subsystem  TreatAsAtomicUnit=on
  VSCP_ComboKey8_enum : Outport
  VSCP_Key8Pass_flg : Outport  Port=2
  wires:
  Data Type Conversion/1 -> [VSCP_ComboKey8_enum]  "VTQD_DiagnosisOff8_enum"
  Delay2/1 -> Maintain/1(Input)
  [VSCP_ComboKey8_enum] -> Delay2/1
  [VSCP_ComboKey8_enum] -> VSCP_ComboKey8_enum/1
  [VSCP_ComboKey8_enum] -> Equal/1
  [VSCP_Key8Pass_flg] -> VSCP_Key8Pass_flg/1
  Equal3/1 -> AND/4
  Delay1/1 -> Equal3/1
  Constant3/1 -> Equal3/2
  [VSCP_ComboKey8_enum] -> Delay1/1
  VSCP_ComboKey7_enum/1 -> [VSCP_ComboKey7_enum]
  OR/1 -> [VSCP_ResetComboKey_flg]  "VSCP_ResetComboKey_flg"
  [VSCP_WriteComboCMD_flg] -> If/2
  [VSCP_ComboKeyCMD_enum] -> Equal1/1
  [VSCP_ComboKeyReset_flg] -> OR/2
  [VSCP_ComboKey7_enum] -> Delay/1
  Equal1/1 -> AND/2
  Constant2/1 -> Equal2/2
  Equal2/1 -> AND/3
  Reset/1(ResetToZero) -> Merge/1
  Merge/1 -> Data Type Conversion/1
  Delay/1 -> Equal2/1
  If/3 -> Maintain/Action
  Constant4/1 -> Equal1/2
  Maintain/1(KeepKey8) -> Merge/3
  Detect Change/1 -> AND/1
  [VSCP_ComboKeyEn_flg] -> Detect Increase/1
  [VSCP_ResetComboKey_flg] -> If/1
  [VSCP_ComboKeyCMD_enum] -> Detect Change/1
  [VSCP_ComboKeyCMD_enum] -> Write/1(Input)
  AND/1 -> [VSCP_WriteComboCMD_flg]  "VSCP_WriteComboCMD_flg"
  Detect Increase/1 -> OR/1
  If/1 -> Reset/Action
  Write/1(WriteCMD) -> Merge/2
  If/2 -> Write/Action
  Constant1/1 -> Equal/2
  Equal/1 -> [VSCP_Key8Pass_flg]  "VTQD_DiagnosisOff8Pass_flg"
  VSCP_ComboKeyCMD_enum/1 -> [VSCP_ComboKeyCMD_enum]
  VSCP_ComboKeyReset_flg/1 -> [VSCP_ComboKeyReset_flg]
  VSCP_ComboKeyEn_flg/1 -> [VSCP_ComboKeyEn_flg]

== system tqd/TQD/TorqueDemand/Signal_convert/SWC2_Subsystem/Big Mike Combo/Combo Key Detection/Engineering Mode/Key1 ==
  VSCP_ComboKeyCMD_enum : Inport
  VSCP_ComboKeyEn_flg : Inport  Port=2
  VSCP_ComboKeyReset_flg : Inport  Port=3
  AND : Logic  Inputs=3  AllPortsSameDT=off  OutDataTypeStr=boolean
  Constant1 : Constant  Value=KTQD_Engineering1_enum
  Constant2 : Constant  Value=ENUM_COMBOKEY_NONE
  Constant4 : Constant  Value=ENUM_COMBOKEY_NONE
  Data Type Conversion : DataTypeConversion  OutDataTypeStr=uint8
  Delay : Delay  DelayLength=1
  Delay1 : Delay  DelayLength=1
  Detect Change : simulink/Logic and Bit Operations/Detect Change  vinit=0  OutDataTypeStr=boolean
  Detect Increase : simulink/Logic and Bit Operations/Detect Increase  vinit=0.0  OutDataTypeStr=boolean
  Equal : RelationalOperator  Operator===  OutDataTypeStr=boolean  RndMeth=Simplest
  Equal1 : RelationalOperator  Operator=~=  OutDataTypeStr=boolean  RndMeth=Simplest
  Equal2 : RelationalOperator  Operator===  OutDataTypeStr=boolean  RndMeth=Simplest
  If : If  NumInputs=2  IfExpression=u1 ~=0  ElseIfExpressions=u2 ~= 0
  Maintain : Subsystem  TreatAsAtomicUnit=on
  Merge : Merge  Inputs=3
  OR : Logic  Operator=OR  AllPortsSameDT=off  OutDataTypeStr=boolean
  Reset : Subsystem  TreatAsAtomicUnit=on
  Write : Subsystem  TreatAsAtomicUnit=on
  VSCP_ComboKey1_enum : Outport
  VSCP_Key1Pass_flg : Outport  Port=2
  wires:
  OR/1 -> [VSCP_ResetComboKey_flg]  "VSCP_ResetComboKey_flg"
  [VSCP_WriteComboCMD_flg] -> If/2
  [VSCP_ComboKeyCMD_enum] -> Equal1/1
  [VSCP_ComboKeyReset_flg] -> OR/2
  [VSCP_ComboKey1_enum] -> Delay/1
  Equal1/1 -> AND/2
  Constant2/1 -> Equal2/2
  Equal2/1 -> AND/3
  Reset/1(ResetToZero) -> Merge/1
  Merge/1 -> Data Type Conversion/1
  Delay/1 -> Equal2/1
  If/3 -> Maintain/Action
  Constant4/1 -> Equal1/2
  Maintain/1(KeepKey1) -> Merge/3
  Detect Change/1 -> AND/1
  [VSCP_ComboKeyEn_flg] -> Detect Increase/1
  [VSCP_ResetComboKey_flg] -> If/1
  [VSCP_ComboKeyCMD_enum] -> Detect Change/1
  [VSCP_ComboKeyCMD_enum] -> Write/1(Input)
  AND/1 -> [VSCP_WriteComboCMD_flg]  "VSCP_WriteComboCMD_flg"
  Detect Increase/1 -> OR/1
  If/1 -> Reset/Action
  Write/1(WriteCMD) -> Merge/2
  If/2 -> Write/Action
  [VSCP_ComboKey1_enum] -> Equal/1
  Constant1/1 -> Equal/2
  Equal/1 -> [VSCP_Key1Pass_flg]  "VTQD_Engineering1Pass_flg"
  VSCP_ComboKeyCMD_enum/1 -> [VSCP_ComboKeyCMD_enum]
  VSCP_ComboKeyReset_flg/1 -> [VSCP_ComboKeyReset_flg]
  VSCP_ComboKeyEn_flg/1 -> [VSCP_ComboKeyEn_flg]
  [VSCP_ComboKey1_enum] -> VSCP_ComboKey1_enum/1
  [VSCP_Key1Pass_flg] -> VSCP_Key1Pass_flg/1
  [VSCP_ComboKey1_enum] -> Delay1/1
  Delay1/1 -> Maintain/1(Input)
  Data Type Conversion/1 -> [VSCP_ComboKey1_enum]  "VTQD_Engineering1_enum"

== system tqd/TQD/TorqueDemand/Signal_convert/SWC2_Subsystem/Big Mike Combo/Combo Key Detection/Engineering Mode/Key2 ==
  VSCP_ComboKeyCMD_enum : Inport
  VSCP_ComboKeyEn_flg : Inport  Port=2
  VSCP_ComboKeyReset_flg : Inport  Port=3
  VSCP_ComboKey1_enum : Inport  Port=4
  AND : Logic  Inputs=4  AllPortsSameDT=off  OutDataTypeStr=boolean
  Constant1 : Constant  Value=KTQD_Engineering2_enum
  Constant2 : Constant  Value=ENUM_COMBOKEY_NONE
  Constant3 : Constant  Value=ENUM_COMBOKEY_NONE
  Constant4 : Constant  Value=ENUM_COMBOKEY_NONE  OutDataTypeStr=uint8
  Data Type Conversion : DataTypeConversion  OutDataTypeStr=uint8
  Delay : Delay  DelayLength=1
  Delay1 : Delay  DelayLength=1
  Delay2 : Delay  DelayLength=1
  Detect Change : simulink/Logic and Bit Operations/Detect Change  vinit=0  OutDataTypeStr=boolean
  Detect Increase : simulink/Logic and Bit Operations/Detect Increase  vinit=0.0  OutDataTypeStr=boolean
  Equal : RelationalOperator  Operator===  OutDataTypeStr=boolean  RndMeth=Simplest
  Equal1 : RelationalOperator  Operator=~=  OutDataTypeStr=boolean  RndMeth=Simplest
  Equal2 : RelationalOperator  Operator=~=  OutDataTypeStr=boolean  RndMeth=Simplest
  Equal3 : RelationalOperator  Operator===  OutDataTypeStr=boolean  RndMeth=Simplest
  If : If  NumInputs=2  IfExpression=u1 ~=0  ElseIfExpressions=u2 ~= 0
  Maintain : Subsystem  TreatAsAtomicUnit=on
  Merge : Merge  Inputs=3
  OR : Logic  Operator=OR  AllPortsSameDT=off  OutDataTypeStr=boolean
  Reset : Subsystem  TreatAsAtomicUnit=on
  Write : Subsystem  TreatAsAtomicUnit=on
  VSCP_ComboKey2_enum : Outport
  VSCP_Key2Pass_flg : Outport  Port=2
  wires:
  [VSCP_Key2Pass_flg] -> VSCP_Key2Pass_flg/1
  [VSCP_ComboKey2_enum] -> VSCP_ComboKey2_enum/1
  VSCP_ComboKeyEn_flg/1 -> [VSCP_ComboKeyEn_flg]
  VSCP_ComboKeyReset_flg/1 -> [VSCP_ComboKeyReset_flg]
  VSCP_ComboKeyCMD_enum/1 -> [VSCP_ComboKeyCMD_enum]
  Equal/1 -> [VSCP_Key2Pass_flg]  "VTQD_Engineering2Pass_flg"
  Constant1/1 -> Equal/2
  [VSCP_ComboKey2_enum] -> Equal/1
  If/2 -> Write/Action
  Write/1(WriteCMD) -> Merge/2
  If/1 -> Reset/Action
  Detect Increase/1 -> OR/1
  AND/1 -> [VSCP_WriteComboCMD_flg]  "VSCP_WriteComboCMD_flg"
  [VSCP_ComboKeyCMD_enum] -> Write/1(Input)
  [VSCP_ComboKeyCMD_enum] -> Detect Change/1
  [VSCP_ResetComboKey_flg] -> If/1
  [VSCP_ComboKeyEn_flg] -> Detect Increase/1
  Detect Change/1 -> AND/1
  Maintain/1(KeepKey2) -> Merge/3
  Constant4/1 -> Equal1/2
  If/3 -> Maintain/Action
  Delay/1 -> Equal2/1
  Merge/1 -> Data Type Conversion/1
  Reset/1(ResetToZero) -> Merge/1
  Equal2/1 -> AND/3
  Constant2/1 -> Equal2/2
  Equal1/1 -> AND/2
  [VSCP_ComboKey1_enum] -> Delay/1
  [VSCP_ComboKeyReset_flg] -> OR/2
  [VSCP_ComboKeyCMD_enum] -> Equal1/1
  [VSCP_WriteComboCMD_flg] -> If/2
  OR/1 -> [VSCP_ResetComboKey_flg]  "VSCP_ResetComboKey_flg"
  VSCP_ComboKey1_enum/1 -> [VSCP_ComboKey1_enum]
  [VSCP_ComboKey2_enum] -> Delay1/1
  Constant3/1 -> Equal3/2
  Delay1/1 -> Equal3/1
  Equal3/1 -> AND/4
  Delay2/1 -> Maintain/1(Input)
  [VSCP_ComboKey2_enum] -> Delay2/1
  Data Type Conversion/1 -> [VSCP_ComboKey2_enum]  "VTQD_Engineering2_enum"

== system tqd/TQD/TorqueDemand/Signal_convert/SWC2_Subsystem/Big Mike Combo/Combo Key Detection/Engineering Mode/Key3 ==
  VSCP_ComboKeyCMD_enum : Inport
  VSCP_ComboKeyEn_flg : Inport  Port=2
  VSCP_ComboKeyReset_flg : Inport  Port=3
  VSCP_ComboKey2_enum : Inport  Port=4
  AND : Logic  Inputs=4  AllPortsSameDT=off  OutDataTypeStr=boolean
  Constant1 : Constant  Value=KTQD_Engineering3_enum
  Constant2 : Constant  Value=ENUM_COMBOKEY_NONE
  Constant3 : Constant  Value=ENUM_COMBOKEY_NONE
  Constant4 : Constant  Value=ENUM_COMBOKEY_NONE
  Data Type Conversion : DataTypeConversion  OutDataTypeStr=uint8
  Delay : Delay  DelayLength=1
  Delay1 : Delay  DelayLength=1
  Delay2 : Delay  DelayLength=1
  Detect Change : simulink/Logic and Bit Operations/Detect Change  vinit=0  OutDataTypeStr=boolean
  Detect Increase : simulink/Logic and Bit Operations/Detect Increase  vinit=0.0  OutDataTypeStr=boolean
  Equal : RelationalOperator  Operator===  OutDataTypeStr=boolean  RndMeth=Simplest
  Equal1 : RelationalOperator  Operator=~=  OutDataTypeStr=boolean  RndMeth=Simplest
  Equal2 : RelationalOperator  Operator=~=  OutDataTypeStr=boolean  RndMeth=Simplest
  Equal3 : RelationalOperator  Operator===  OutDataTypeStr=boolean  RndMeth=Simplest
  If : If  NumInputs=2  IfExpression=u1 ~=0  ElseIfExpressions=u2 ~= 0
  Maintain : Subsystem  TreatAsAtomicUnit=on
  Merge : Merge  Inputs=3
  OR : Logic  Operator=OR  AllPortsSameDT=off  OutDataTypeStr=boolean
  Reset : Subsystem  TreatAsAtomicUnit=on
  Write : Subsystem  TreatAsAtomicUnit=on
  VSCP_ComboKey3_enum : Outport
  VSCP_Key3Pass_flg : Outport  Port=2
  wires:
  VSCP_ComboKey2_enum/1 -> [VSCP_ComboKey2_enum]
  OR/1 -> [VSCP_ResetComboKey_flg]  "VSCP_ResetComboKey_flg"
  [VSCP_WriteComboCMD_flg] -> If/2
  [VSCP_ComboKeyCMD_enum] -> Equal1/1
  [VSCP_ComboKeyReset_flg] -> OR/2
  [VSCP_ComboKey2_enum] -> Delay/1
  Equal1/1 -> AND/2
  Constant2/1 -> Equal2/2
  Equal2/1 -> AND/3
  Reset/1(ResetToZero) -> Merge/1
  Merge/1 -> Data Type Conversion/1
  Delay/1 -> Equal2/1
  If/3 -> Maintain/Action
  Constant4/1 -> Equal1/2
  Maintain/1(KeepKey3) -> Merge/3
  Detect Change/1 -> AND/1
  [VSCP_ComboKeyEn_flg] -> Detect Increase/1
  [VSCP_ResetComboKey_flg] -> If/1
  [VSCP_ComboKeyCMD_enum] -> Detect Change/1
  [VSCP_ComboKeyCMD_enum] -> Write/1(Input)
  AND/1 -> [VSCP_WriteComboCMD_flg]  "VSCP_WriteComboCMD_flg"
  Detect Increase/1 -> OR/1
  If/1 -> Reset/Action
  Write/1(WriteCMD) -> Merge/2
  If/2 -> Write/Action
  Constant1/1 -> Equal/2
  Equal/1 -> [VSCP_Key3Pass_flg]  "VTQD_Engineering3Pass_flg"
  VSCP_ComboKeyCMD_enum/1 -> [VSCP_ComboKeyCMD_enum]
  VSCP_ComboKeyReset_flg/1 -> [VSCP_ComboKeyReset_flg]
  VSCP_ComboKeyEn_flg/1 -> [VSCP_ComboKeyEn_flg]
  [VSCP_ComboKey3_enum] -> VSCP_ComboKey3_enum/1
  [VSCP_ComboKey3_enum] -> Equal/1
  [VSCP_Key3Pass_flg] -> VSCP_Key3Pass_flg/1
  Delay1/1 -> Equal3/1
  Equal3/1 -> AND/4
  Constant3/1 -> Equal3/2
  [VSCP_ComboKey3_enum] -> Delay1/1
  Delay2/1 -> Maintain/1(Input)
  [VSCP_ComboKey3_enum] -> Delay2/1
  Data Type Conversion/1 -> [VSCP_ComboKey3_enum]  "VTQD_Engineering3_enum"

== system tqd/TQD/TorqueDemand/Signal_convert/SWC2_Subsystem/Big Mike Combo/Combo Key Detection/Engineering Mode/Key4 ==
  VSCP_ComboKeyCMD_enum : Inport
  VSCP_ComboKeyEn_flg : Inport  Port=2
  VSCP_ComboKeyReset_flg : Inport  Port=3
  VSCP_ComboKey3_enum : Inport  Port=4
  AND : Logic  Inputs=4  AllPortsSameDT=off  OutDataTypeStr=boolean
  Constant1 : Constant  Value=KTQD_Engineering4_enum
  Constant2 : Constant  Value=ENUM_COMBOKEY_NONE
  Constant3 : Constant  Value=ENUM_COMBOKEY_NONE
  Constant4 : Constant  Value=ENUM_COMBOKEY_NONE
  Data Type Conversion : DataTypeConversion  OutDataTypeStr=uint8
  Delay : Delay  DelayLength=1
  Delay1 : Delay  DelayLength=1
  Delay2 : Delay  DelayLength=1
  Detect Change : simulink/Logic and Bit Operations/Detect Change  vinit=0  OutDataTypeStr=boolean
  Detect Increase : simulink/Logic and Bit Operations/Detect Increase  vinit=0.0  OutDataTypeStr=boolean
  Equal : RelationalOperator  Operator===  OutDataTypeStr=boolean  RndMeth=Simplest
  Equal1 : RelationalOperator  Operator=~=  OutDataTypeStr=boolean  RndMeth=Simplest
  Equal2 : RelationalOperator  Operator=~=  OutDataTypeStr=boolean  RndMeth=Simplest
  Equal3 : RelationalOperator  Operator===  OutDataTypeStr=boolean  RndMeth=Simplest
  If : If  NumInputs=2  IfExpression=u1 ~=0  ElseIfExpressions=u2 ~= 0
  Maintain : Subsystem  TreatAsAtomicUnit=on
  Merge : Merge  Inputs=3
  OR : Logic  Operator=OR  AllPortsSameDT=off  OutDataTypeStr=boolean
  Reset : Subsystem  TreatAsAtomicUnit=on
  Write : Subsystem  TreatAsAtomicUnit=on
  VSCP_ComboKey4_enum : Outport
  VSCP_Key4Pass_flg : Outport  Port=2
  wires:
  [VSCP_ComboKey4_enum] -> Equal/1
  VSCP_ComboKeyEn_flg/1 -> [VSCP_ComboKeyEn_flg]
  VSCP_ComboKeyReset_flg/1 -> [VSCP_ComboKeyReset_flg]
  VSCP_ComboKeyCMD_enum/1 -> [VSCP_ComboKeyCMD_enum]
  Equal/1 -> [VSCP_Key4Pass_flg]  "VTQD_Engineering4Pass_flg"
  Constant1/1 -> Equal/2
  If/2 -> Write/Action
  Write/1(WriteCMD) -> Merge/2
  If/1 -> Reset/Action
  Detect Increase/1 -> OR/1
  AND/1 -> [VSCP_WriteComboCMD_flg]  "VSCP_WriteComboCMD_flg"
  [VSCP_ComboKeyCMD_enum] -> Write/1(Input)
  [VSCP_ComboKeyCMD_enum] -> Detect Change/1
  [VSCP_ResetComboKey_flg] -> If/1
  [VSCP_ComboKeyEn_flg] -> Detect Increase/1
  Detect Change/1 -> AND/1
  Maintain/1(KeepKey4) -> Merge/3
  Constant4/1 -> Equal1/2
  If/3 -> Maintain/Action
  Delay/1 -> Equal2/1
  Merge/1 -> Data Type Conversion/1
  Reset/1(ResetToZero) -> Merge/1
  Equal2/1 -> AND/3
  Constant2/1 -> Equal2/2
  Equal1/1 -> AND/2
  [VSCP_ComboKey3_enum] -> Delay/1
  [VSCP_ComboKeyReset_flg] -> OR/2
  [VSCP_ComboKeyCMD_enum] -> Equal1/1
  [VSCP_WriteComboCMD_flg] -> If/2
  OR/1 -> [VSCP_ResetComboKey_flg]  "VSCP_ResetComboKey_flg"
  VSCP_ComboKey3_enum/1 -> [VSCP_ComboKey3_enum]
  [VSCP_ComboKey4_enum] -> Delay1/1
  Constant3/1 -> Equal3/2
  Delay1/1 -> Equal3/1
  Equal3/1 -> AND/4
  [VSCP_Key4Pass_flg] -> VSCP_Key4Pass_flg/1
  [VSCP_ComboKey4_enum] -> VSCP_ComboKey4_enum/1
  [VSCP_ComboKey4_enum] -> Delay2/1
  Delay2/1 -> Maintain/1(Input)
  Data Type Conversion/1 -> [VSCP_ComboKey4_enum]  "VTQD_Engineering4_enum"
